simulink model "AOCS_m"  (R2023b)
settings: Solver=VariableStepAuto  StartTime=0.0  StopTime=100  MaxStep=0.01  RelTol=1e-4  AbsTol=1e-5
libraries: autolibbldc x3
settings Model: SimulationMode=accelerator  Creator=tiwan  LastModifiedBy=tiwan
settings SolverCC: AutoScaleAbsTol=off  InitialStep=0.01  ZeroCrossControl=EnableAll

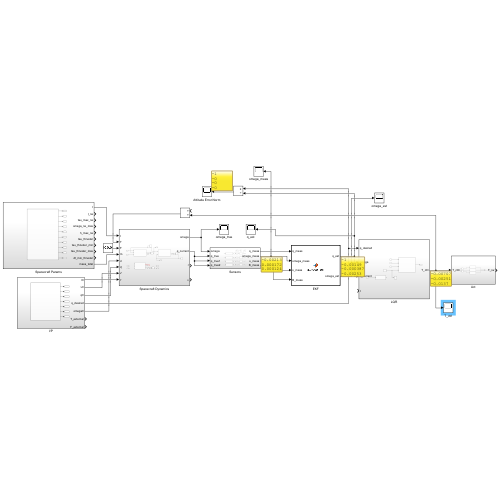
[thumbnail: Simulink's stored preview of the top-level diagram]
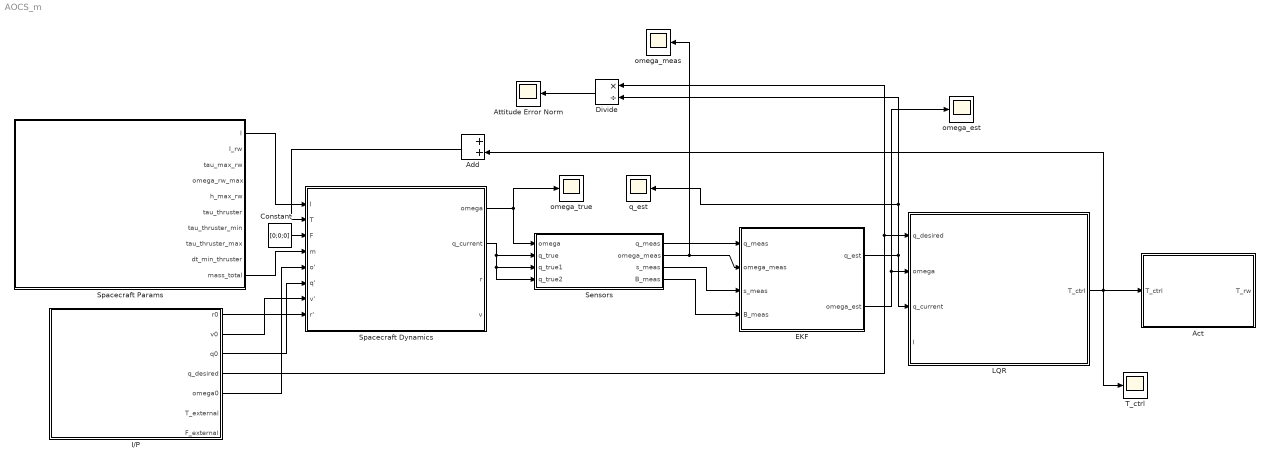
== system AOCS_m ==
  Act : Subsystem
  Add : Sum
  Attitude Error Norm : Scope
  Constant : Constant  Value=[0;0;0]
  Divide : Product  Inputs=*/
  EKF : MATLAB Function  TreatAsAtomicUnit=on
  I/P : Subsystem
  LQR : Subsystem
  Sensors : Subsystem
  Spacecraft Dynamics : Subsystem
  Spacecraft Params : Subsystem
  T_ctrl : Scope
  omega_est : Scope
  omega_meas : Scope
  omega_true : Scope
  q_est : Scope
  wires:
  Spacecraft Params/1(I) -> Spacecraft Dynamics/1(I)
  I/P/1(r0) -> Spacecraft Dynamics/8(r')
  I/P/2(v0) -> Spacecraft Dynamics/7(v')
  I/P/3(q0) -> Spacecraft Dynamics/6(q')
  I/P/5(omega0) -> Spacecraft Dynamics/5(o')
  I/P/4(q_desired) -> LQR/1(q_desired), Divide/1
  Spacecraft Dynamics/1(omega) -> Sensors/1(omega), omega_true/1
  Spacecraft Dynamics/2(q_current) -> Sensors/4(q_true2), Sensors/3(q_true1), Sensors/2(q_true)
  LQR/1(T_ctrl) -> Add/2, T_ctrl/1, Act/1(T_ctrl)
  Sensors/2(omega_meas) -> EKF/2(omega_meas), omega_meas/1
  Sensors/1(q_meas) -> EKF/1(q_meas)
  Sensors/3(s_meas) -> EKF/3(s_meas)
  Sensors/4(B_meas) -> EKF/4(B_meas)
  EKF/1(q_est) -> Divide/2, q_est/1, LQR/3(q_current)
  EKF/2(omega_est) -> LQR/2(omega), omega_est/1
  Spacecraft Params/10(mass_total) -> Spacecraft Dynamics/4(m)
  Constant/1 -> Spacecraft Dynamics/3(F)
  Divide/1 -> Attitude Error Norm/1
  Add/1 -> Spacecraft Dynamics/2(T)

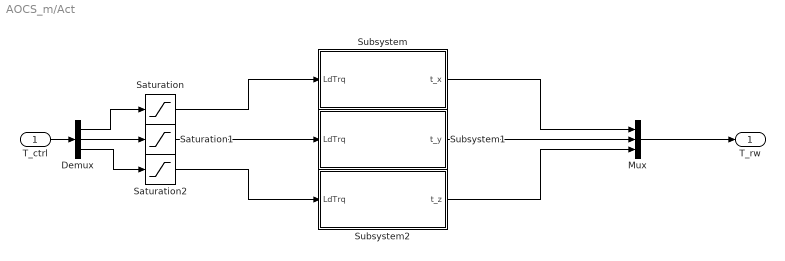
== system AOCS_m/Act ==
  T_ctrl : Inport
  Demux : Demux  Outputs=3
  Mux : Mux  Inputs=3
  Saturation : Saturate  UpperLimit=0.2  LowerLimit=-0.2
  Saturation1 : Saturate  UpperLimit=0.2  LowerLimit=-0.2
  Saturation2 : Saturate  UpperLimit=0.2  LowerLimit=-0.2
  Subsystem : Subsystem
  Subsystem1 : Subsystem
  Subsystem2 : Subsystem
  T_rw : Outport
  wires:
  T_ctrl/1 -> Demux/1
  Demux/1 -> Saturation/1
  Demux/2 -> Saturation1/1
  Demux/3 -> Saturation2/1
  Mux/1 -> T_rw/1
  Saturation/1 -> Subsystem/1(LdTrq)
  Saturation1/1 -> Subsystem1/1(LdTrq)
  Saturation2/1 -> Subsystem2/1(LdTrq)
  Subsystem1/1(t_y) -> Mux/2
  Subsystem/1(t_x) -> Mux/1
  Subsystem2/1(t_z) -> Mux/3

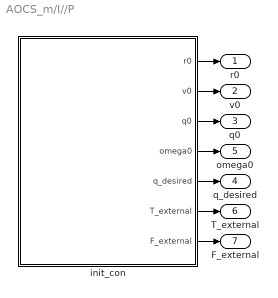
== system AOCS_m/I//P ==
  init_con : MATLAB Function  TreatAsAtomicUnit=on
  r0 : Outport
  v0 : Outport  Port=2
  q0 : Outport  Port=3
  q_desired : Outport  Port=4
  omega0 : Outport  Port=5
  T_external : Outport  Port=6
  F_external : Outport  Port=7
  wires:
  init_con/1(r0) -> r0/1
  init_con/7(F_external) -> F_external/1
  init_con/6(T_external) -> T_external/1
  init_con/5(q_desired) -> q_desired/1
  init_con/2(v0) -> v0/1
  init_con/3(q0) -> q0/1
  init_con/4(omega0) -> omega0/1

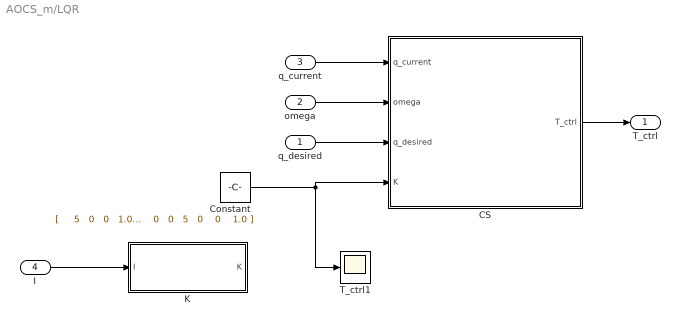
== system AOCS_m/LQR ==
  q_desired : Inport
  omega : Inport  Port=2
  q_current : Inport  Port=3
  I : Inport  Port=4
  CS : MATLAB Function  TreatAsAtomicUnit=on
  Constant : Constant  Value=|
      | [
      |     5   0   0   1.0  0    0;
      |     0   5   0   0    1.0  0;
      |     0   0   5   0    0    1.0
      | ]
  K : MATLAB Function  TreatAsAtomicUnit=on
  T_ctrl1 : Scope
  T_ctrl : Outport
  wires:
  q_desired/1 -> CS/3(q_desired)
  omega/1 -> CS/2(omega)
  q_current/1 -> CS/1(q_current)
  CS/1(T_ctrl) -> T_ctrl/1
  I/1 -> K/1(I)
  Constant/1 -> CS/4(K), T_ctrl1/1

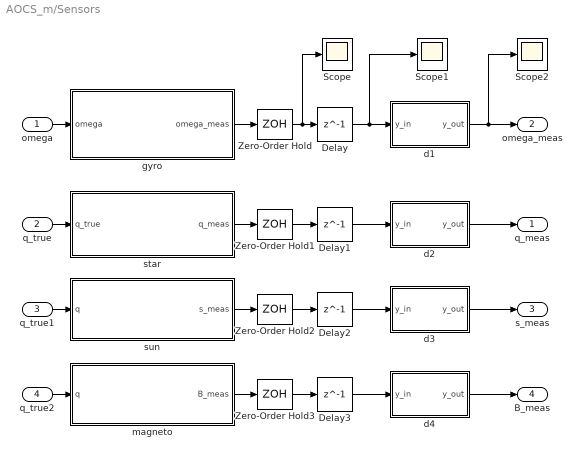
== system AOCS_m/Sensors ==
  omega : Inport
  q_true : Inport  Port=2
  q_true1 : Inport  Port=3
  q_true2 : Inport  Port=4
  Delay{,1..3} (4 alike) : Delay  DelayLength=1  InitialCondition=0  SampleTime=0.05
  Scope : Scope
  Scope1 : Scope
  Scope2 : Scope
  Zero-Order Hold : ZeroOrderHold  SampleTime=0.1
  Zero-Order Hold1 : ZeroOrderHold  SampleTime=-1
  Zero-Order Hold2 : ZeroOrderHold  SampleTime=-1
  Zero-Order Hold3 : ZeroOrderHold  SampleTime=-1
  d1 : MATLAB Function  TreatAsAtomicUnit=on
  d2 : MATLAB Function  TreatAsAtomicUnit=on
  d3 : MATLAB Function  TreatAsAtomicUnit=on
  d4 : MATLAB Function  TreatAsAtomicUnit=on
  gyro : MATLAB Function  TreatAsAtomicUnit=on
  magneto : MATLAB Function  TreatAsAtomicUnit=on
  star : MATLAB Function  TreatAsAtomicUnit=on
  sun : MATLAB Function  TreatAsAtomicUnit=on
  q_meas : Outport
  omega_meas : Outport  Port=2
  s_meas : Outport  Port=3
  B_meas : Outport  Port=4
  wires:
  omega/1 -> gyro/1(omega)
  q_true/1 -> star/1(q_true)
  star/1(q_meas) -> Zero-Order Hold1/1
  gyro/1(omega_meas) -> Zero-Order Hold/1
  Zero-Order Hold/1 -> Scope/1, Delay/1
  Zero-Order Hold1/1 -> Delay1/1
  Delay/1 -> Scope1/1, d1/1(y_in)
  Delay1/1 -> d2/1(y_in)
  d2/1(y_out) -> q_meas/1
  q_true1/1 -> sun/1(q)
  q_true2/1 -> magneto/1(q)
  magneto/1(B_meas) -> Zero-Order Hold3/1
  sun/1(s_meas) -> Zero-Order Hold2/1
  Zero-Order Hold2/1 -> Delay2/1
  Zero-Order Hold3/1 -> Delay3/1
  Delay2/1 -> d3/1(y_in)
  Delay3/1 -> d4/1(y_in)
  d3/1(y_out) -> s_meas/1
  d4/1(y_out) -> B_meas/1
  d1/1(y_out) -> Scope2/1, omega_meas/1

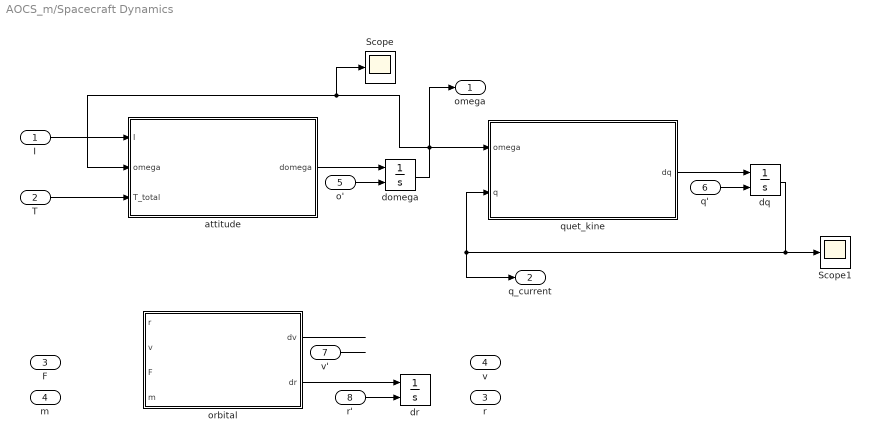
== system AOCS_m/Spacecraft Dynamics ==
  I : Inport
  T : Inport  Port=2
  F : Inport  Port=3
  m : Inport  Port=4
  o' : Inport  Port=5
  q' : Inport  Port=6
  v' : Inport  Port=7
  r' : Inport  Port=8
  Scope : Scope
  Scope1 : Scope
  attitude : MATLAB Function  TreatAsAtomicUnit=on
  domega : Integrator  InitialConditionSource=external
  dq : Integrator  InitialConditionSource=external
  dr : Integrator  InitialConditionSource=external
  orbital : MATLAB Function  TreatAsAtomicUnit=on
  quet_kine : MATLAB Function  TreatAsAtomicUnit=on
  omega : Outport
  q_current : Outport  Port=2
  r : Outport  Port=3
  v : Outport  Port=4
  wires:
  attitude/1(domega) -> domega/1
  domega/1 -> omega/1, Scope/1, attitude/2(omega), quet_kine/1(omega)
  quet_kine/1(dq) -> dq/1
  dq/1 -> Scope1/1, quet_kine/2(q), q_current/1
  orbital/1(dv) -> ?
  orbital/2(dr) -> dr/1
  I/1 -> attitude/1(I)
  T/1 -> attitude/3(T_total)
  o'/1 -> domega/2
  q'/1 -> dq/2
  v'/1 -> ?
  r'/1 -> dr/2

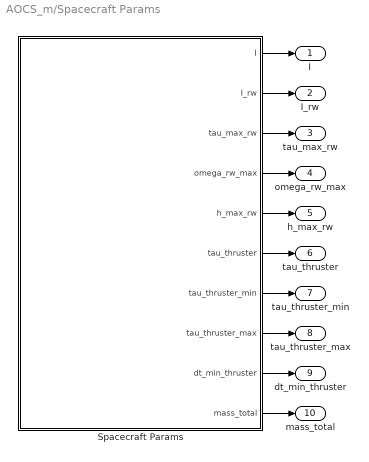
== system AOCS_m/Spacecraft Params ==
  Spacecraft Params : MATLAB Function  TreatAsAtomicUnit=on
  I : Outport
  I_rw : Outport  Port=2
  tau_max_rw : Outport  Port=3
  omega_rw_max : Outport  Port=4
  h_max_rw : Outport  Port=5
  tau_thruster : Outport  Port=6
  tau_thruster_min : Outport  Port=7
  tau_thruster_max : Outport  Port=8
  dt_min_thruster : Outport  Port=9
  mass_total : Outport  Port=10
  wires:
  Spacecraft Params/1(I) -> I/1
  Spacecraft Params/2(I_rw) -> I_rw/1
  Spacecraft Params/3(tau_max_rw) -> tau_max_rw/1
  Spacecraft Params/4(omega_rw_max) -> omega_rw_max/1
  Spacecraft Params/5(h_max_rw) -> h_max_rw/1
  Spacecraft Params/6(tau_thruster) -> tau_thruster/1
  Spacecraft Params/7(tau_thruster_min) -> tau_thruster_min/1
  Spacecraft Params/8(tau_thruster_max) -> tau_thruster_max/1
  Spacecraft Params/9(dt_min_thruster) -> dt_min_thruster/1
  Spacecraft Params/10(mass_total) -> mass_total/1

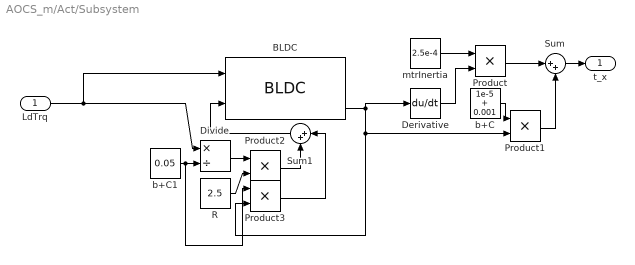
== system AOCS_m/Act/Subsystem ==
  LdTrq : Inport
  BLDC : autolibbldc/BLDC  VariantControl=pmsmVariant==pmsmEnum.TorqueInput  MechInput=Torque  SimType=Continuous  BlockSampleTime=25e-6  p=1  Rs=2.5  Ld=0.005  Lq=0.005  Lambda=0.0064  J=2.5e-4  B=2.6369e-06  F=0  Id_init=0  Iq_init=0  Th_init=0  Omega_init=0  RefBlkName='autolibbldc/BLDC'  aMode=5
      settings: LibrarySourceBlock=mcblib/Electrical Systems/Motors/BLDC
  Derivative : Derivative
  Divide : Product  Inputs=*/
  Product{,1..3} (4 alike) : Product
  R : Constant  Value=2.5
  Sum : Sum  Inputs=|++
  Sum1 : Sum  Inputs=|++
  b+C : Constant  Value=1e-5 + 0.001
  b+C1 : Constant  Value=0.05
  mtrInertia : Constant  Value=2.5e-4
  t_x : Outport
  wires:
  Product3/1 -> Sum1/1
  b+C1/1 -> Product3/1, Divide/2
  BLDC/3 -> Product3/2, Product1/2, Derivative/1
  LdTrq/1 -> Divide/1, BLDC/1
  R/1 -> Product2/2
  b+C/1 -> Product1/1
  Derivative/1 -> Product/2
  Sum1/1 -> BLDC/2
  mtrInertia/1 -> Product/1
  Product/1 -> Sum/1
  Divide/1 -> Product2/1
  Product1/1 -> Sum/2
  Product2/1 -> Sum1/2
  Sum/1 -> t_x/1

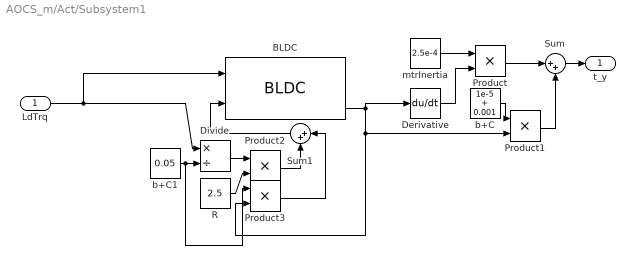
== system AOCS_m/Act/Subsystem1 ==
  LdTrq : Inport
  BLDC : autolibbldc/BLDC  VariantControl=pmsmVariant==pmsmEnum.TorqueInput  MechInput=Torque  SimType=Continuous  BlockSampleTime=25e-6  p=1  Rs=2.5  Ld=0.005  Lq=0.005  Lambda=0.0064  J=2.5e-4  B=2.6369e-06  F=0  Id_init=0  Iq_init=0  Th_init=0  Omega_init=0  RefBlkName='autolibbldc/BLDC'  aMode=5
      settings: LibrarySourceBlock=mcblib/Electrical Systems/Motors/BLDC
  Derivative : Derivative
  Divide : Product  Inputs=*/
  Product{,1..3} (4 alike) : Product
  R : Constant  Value=2.5
  Sum : Sum  Inputs=|++
  Sum1 : Sum  Inputs=|++
  b+C : Constant  Value=1e-5 + 0.001
  b+C1 : Constant  Value=0.05
  mtrInertia : Constant  Value=2.5e-4
  t_y : Outport
  wires:
  Product3/1 -> Sum1/1
  b+C1/1 -> Product3/1, Divide/2
  BLDC/3 -> Product3/2, Product1/2, Derivative/1
  LdTrq/1 -> Divide/1, BLDC/1
  R/1 -> Product2/2
  b+C/1 -> Product1/1
  Derivative/1 -> Product/2
  Sum1/1 -> BLDC/2
  mtrInertia/1 -> Product/1
  Product/1 -> Sum/1
  Divide/1 -> Product2/1
  Product1/1 -> Sum/2
  Product2/1 -> Sum1/2
  Sum/1 -> t_y/1

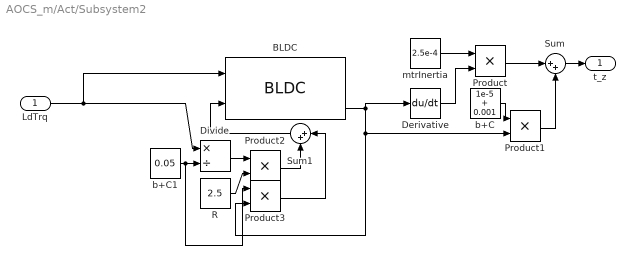
== system AOCS_m/Act/Subsystem2 ==
  LdTrq : Inport
  BLDC : autolibbldc/BLDC  VariantControl=pmsmVariant==pmsmEnum.TorqueInput  MechInput=Torque  SimType=Continuous  BlockSampleTime=25e-6  p=1  Rs=2.5  Ld=0.005  Lq=0.005  Lambda=0.0064  J=2.5e-4  B=2.6369e-06  F=0  Id_init=0  Iq_init=0  Th_init=0  Omega_init=0  RefBlkName='autolibbldc/BLDC'  aMode=5
      settings: LibrarySourceBlock=mcblib/Electrical Systems/Motors/BLDC
  Derivative : Derivative
  Divide : Product  Inputs=*/
  Product{,1..3} (4 alike) : Product
  R : Constant  Value=2.5
  Sum : Sum  Inputs=|++
  Sum1 : Sum  Inputs=|++
  b+C : Constant  Value=1e-5 + 0.001
  b+C1 : Constant  Value=0.05
  mtrInertia : Constant  Value=2.5e-4
  t_z : Outport
  wires:
  Product3/1 -> Sum1/1
  b+C1/1 -> Product3/1, Divide/2
  BLDC/3 -> Product3/2, Product1/2, Derivative/1
  LdTrq/1 -> Divide/1, BLDC/1
  R/1 -> Product2/2
  b+C/1 -> Product1/1
  Derivative/1 -> Product/2
  Sum1/1 -> BLDC/2
  mtrInertia/1 -> Product/1
  Product/1 -> Sum/1
  Divide/1 -> Product2/1
  Product1/1 -> Sum/2
  Product2/1 -> Sum1/2
  Sum/1 -> t_z/1

== matlab function AOCS_m/Sensors/d2 ==
  data: y_in input; y_out output
function y_out = dropout(y_in)
% Simulate dropout with 2% chance
if rand < 0.02
    y_out = zeros(size(y_in));  % Lost reading
else
    y_out = y_in;
end
end

== matlab function AOCS_m/Sensors/sun ==
  settings: updateMethod=DISCRETE
  data: q input; s_meas output
function s_meas = sun_sensor(q)
% Constants
s_inertial = [-1; 0; 0];           % Sun vector in inertial frame (unit vector)
noise_std = 0.01;                  % Sun sensor noise

% Convert quaternion to rotation matrix
q0 = q(1); qv = q(2:4);
q_cross = [    0   -qv(3)  qv(2);
            qv(3)     0   -qv(1);
           -qv(2)  qv(1)     0 ];
R = (q0^2 - qv' * qv) * eye(3) + 2 * (qv * qv') - 2 * q0 * q_cross;

% Transform Sun vector to body frame
s_body = R * s_inertial;

% Add noise
s_meas = s_body + noise_std * randn(3,1);
end

== matlab function AOCS_m/Sensors/magneto ==
  settings: updateMethod=DISCRETE
  data: q input; B_meas output
function B_meas = magnetometer(q)
% Constants
B_inertial = [0.2; -0.3; 0.4];     % Earth's magnetic field in inertial frame (μT)
noise_std = 0.01;                  % Magnetometer noise

% Convert quaternion to rotation matrix
q0 = q(1); qv = q(2:4);
q_cross = [    0   -qv(3)  qv(2);
            qv(3)     0   -qv(1);
           -qv(2)  qv(1)     0 ];
R = (q0^2 - qv' * qv) * eye(3) + 2 * (qv * qv') - 2 * q0 * q_cross;

% Transform magnetic field vector to body frame
B_body = R * B_inertial;

% Add noise
B_meas = B_body + noise_std * randn(3,1);
end

== matlab function AOCS_m/EKF ==
  data: q_meas input; q_est output; omega_meas input; s_meas input; B_meas input; omega_est output
function [q_est, omega_est] = attitude_ekf(q_meas, omega_meas, s_meas, B_meas)

% ======= Input Guards =======
if isempty(q_meas) || norm(q_meas) == 0 || any(isnan(q_meas))
    q_meas = [1; 0; 0; 0];  % fallback to identity quaternion
end

if isempty(omega_meas) || any(isnan(omega_meas))
    omega_meas = [0; 0; 0];
end

% ======= Persistent Variables =======
persistent x P
dt = 0.01;

if isempty(x)
    x = [q_meas; omega_meas];     % Initial state
    P = 1e-2 * eye(7);             % Initial covariance
end

% ======= Prediction Step =======
q = x(1:4);
omega = x(5:7);

% Quaternion derivative using Omega matrix
Omega = [0, -omega';
         omega, -skew(omega)];

q_dot = 0.5 * Omega * q;
q_pred = q + dt * q_dot;

% Normalize prediction
if norm(q_pred) == 0 || any(isnan(q_pred))
    q_pred = [1; 0; 0; 0];
else
    q_pred = q_pred / norm(q_pred);
end

omega_pred = omega;

% Jacobians (simplified)
F = eye(7);
Q = 1e-4 * eye(7);

x_pred = [q_pred; omega_pred];
P = F * P * F' + Q;

% ======= Measurement Update =======
H = eye(7);                 % Direct observation
R = 1e-3 * eye(7);           % Measurement noise

z = [q_meas; omega_meas];  % Measurement vector
z_pred = x_pred;           % Predicted measurement

% Kalman Gain
K = P * H' / (H * P * H' + R);

% EKF Update
x = x_pred + K * (z - z_pred);

% Normalize quaternion again
if norm(x(1:4)) == 0 || any(isnan(x(1:4)))
    x(1:4) = [1; 0; 0; 0];
else
    x(1:4) = x(1:4) / norm(x(1:4));
end

P = (eye(7) - K * H) * P;

% ======= Outputs =======
q_est = x(1:4);
omega_est = x(5:7);

end

% ======= Helper Function =======
function S = skew(w)
S = [ 0    -w(3)  w(2);
      w(3)  0    -w(1);
     -w(2)  w(1)  0   ];
end

== matlab function AOCS_m/Sensors/d3 ==
  data: y_in input; y_out output
function y_out = dropout(y_in)
% Simulate dropout with 2% chance
if rand < 0.02
    y_out = zeros(size(y_in));  % Lost reading
else
    y_out = y_in;
end
end

== matlab function AOCS_m/Sensors/d4 ==
  data: y_in input; y_out output
function y_out = dropout(y_in)
% Simulate dropout with 2% chance
if rand < 0.02
    y_out = zeros(size(y_in));  % Lost reading
else
    y_out = y_in;
end
end

== matlab function AOCS_m/LQR/K ==
  data: K output; I input
function K = computeK_manual(I)
% Fully Simulink-compatible LQR gain using Riccati iteration, no inv()

% Output definition
K = zeros(3,6);

% Validate input inertia
if any(size(I) ~= [3, 3])
    return;
end

% A, B matrices
A = [zeros(3), 0.5 * eye(3);
     zeros(3), zeros(3)];
B = [zeros(3);
     I \ eye(3)];  % Same as inv(I) * I_identity

% LQR weights
Q = diag([100, 100, 100, 5, 5, 5]);
R = 0.1 * eye(3);

% Riccati gradient descent
S = Q;
alpha = 1e-3;
max_iter = 500;
tol = 1e-4;

for i = 1:max_iter
    BT_S = B' * S;
    E = A' * S + S * A - S * B * (R \ BT_S) + Q;
    
    if norm(E, 'fro') < tol
        break;
    end
    
    S = S - alpha * E;
end

% Final LQR gain
K = R \ (B' * S);
end

== matlab function AOCS_m/Spacecraft Dynamics/attitude ==
  data: I input; domega output; omega input; T_total input
function domega = angular_dynamics(I, omega, T_total)
% Safety checks
if any(isnan(omega)) || any(isinf(omega))
    omega = [0;0;0];
end
if any(isnan(T_total)) || any(isinf(T_total))
    T_total = [0;0;0];
end

omega_cross = [  0        -omega(3)  omega(2);
              omega(3)     0       -omega(1);
             -omega(2)  omega(1)     0    ];

% Prevent singular matrix issues
if det(I) < 1e-6
    I = I + 1e-3 * eye(3);  % Regularize inertia
end

domega = I \ (T_total - omega_cross * (I * omega));
end

== matlab function AOCS_m/Spacecraft Params/Spacecraft Params ==
  data: I output; I_rw output; tau_max_rw output; omega_rw_max output; h_max_rw output; tau_thruster output; tau_thruster_min output; tau_thruster_max output; dt_min_thruster output; mass_total output
function [I, I_rw, tau_max_rw, omega_rw_max, h_max_rw, ...
          tau_thruster, tau_thruster_min, tau_thruster_max, ...
          dt_min_thruster, mass_total] = spacecraft_parameters()

% Spacecraft Moment of Inertia (kg·m²)
I = diag([2.5, 2.0, 1.8]);  % Customize per spacecraft

% Reaction Wheel Parameters
I_rw = [0.02; 0.02; 0.02];                    % Reaction wheel inertias
tau_max_rw = [0.1; 0.1; 0.1];                 % Max torque per RW (Nm)
omega_rw_max = [6000; 6000; 6000] * 2*pi/60;                  % Max RW speed (rad/s)
h_max_rw = I_rw .* omega_rw_max;             % Max angular momentum storage

% Thruster Parameters
tau_thruster = [0; 0; 0.5];      % Constant torque or command placeholder
tau_thruster_min = 0.01;         % Minimum on-time torque (Nm)
tau_thruster_max = 1.0;          % Max safe torque (Nm)
dt_min_thruster = 0.1;           % Min pulse time (s)

% Spacecraft Total Mass
mass_total = 50;  % kg

end

== matlab function AOCS_m/Spacecraft Dynamics/quet_kine ==
  data: omega input; dq output; q input
function dq = quaternion_kinematics(omega, q)
% omega: angular velocity [3x1]
% q: current quaternion [4x1]

Omega = [0       -omega(1) -omega(2) -omega(3);
         omega(1)  0        omega(3) -omega(2);
         omega(2) -omega(3) 0         omega(1);
         omega(3) omega(2) -omega(1)  0];

dq = 0.5 * Omega * q;
end

== matlab function AOCS_m/Spacecraft Dynamics/orbital ==
  data: r input; dv output; v input; F input; m input; dr output
function [dv, dr] = orbital_dynamics(r, v, F, m)
% r: position vector [3x1]
% v: velocity vector [3x1]
% F: total force applied [3x1]
% m: spacecraft mass (scalar)

mu = 398600.4418;  % Earth's gravitational parameter, km^3/s^2

% Two-body gravity + applied force
r_norm = norm(r);
a_gravity = -mu * r / r_norm^3;
a_applied = F / m;

dv = a_gravity + a_applied;
dr = v;
end

== matlab function AOCS_m/I//P/init_con ==
  data: r0 output; v0 output; q0 output; omega0 output; q_desired output; T_external output; F_external output
function [r0, v0, q0, omega0, q_desired, T_external, F_external] = initial_conditions()

% Initial orbital position (e.g., 700 km circular orbit in ECI frame)
r0 = [7000; 0; 0];          % km
v0 = [0; 7.5; 0];           % km/s (rough circular speed)

% Initial attitude (slightly off identity quaternion)
q0 = [0.999; 0.01; 0.01; 0.01];  % Should be normalized

% Initial angular velocity (rad/s)
omega0 = [0.01; 0.005; -0.01];   % Small rotation rate

% Desired attitude
q_desired = [1; 0; 0; 0];  % No rotation (identity quaternion)

% External disturbance torque (Nm)
T_external = [0.0001; 0.0001; 0.0002];

% External force (e.g., drag, solar radiation pressure) (N)
F_external = [0; 0; 0];  % Start with 0, can be added later

end

== matlab function AOCS_m/LQR/CS ==
  data: q_current input; T_ctrl output; omega input; q_desired input; K input
function T_ctrl = lqr_attitude_control(q_current, omega,q_desired, K)
% Inputs:
%   q_current: [4x1] current quaternion
%   omega:     [3x1] angular velocity
%   q_desired: [4x1] desired quaternion
%   K:         [3x6] LQR gain matrix

% Normalize quaternions (important for numerical stability)
q_current = q_current / norm(q_current);
q_desired = q_desired / norm(q_desired);

% Quaternion error: q_err = q_desired ⊗ q_current⁻¹
q_conj = [q_current(1); -q_current(2:4)];
q_err = quatmultiply(q_desired', q_conj')';  % result is 4x1

% Use only vector part of q_err (proportional part)
delta_q = q_err(2:4);  % 3x1

% LQR control law
x = [delta_q; omega];    % 6x1
T_ctrl = -K * x;         % 3x1 torque output

end

== matlab function AOCS_m/Sensors/gyro ==
  settings: updateMethod=DISCRETE
  data: omega input; omega_meas output
function omega_meas = gyro_sensor(omega)
% Simple gyroscope with bias and Gaussian noise
bias = [0.0005; -0.0003; 0.0004];     % Constant bias (rad/s)
noise_std = 0.001;                    % Noise std dev (rad/s)

omega_meas = omega + bias + noise_std * randn(3,1);
end

== matlab function AOCS_m/Sensors/star ==
  settings: updateMethod=DISCRETE
  data: q_true input; q_meas output
function q_meas = star_tracker(q_true)
% Star tracker with small attitude noise
noise_std = 0.002;

q_meas = q_true + noise_std * randn(4,1);
q_meas = q_meas / norm(q_meas);  % Normalize to unit quaternion
end

== matlab function AOCS_m/Sensors/d1 ==
  data: y_in input; y_out output
function y_out = dropout(y_in)
% Simulate dropout with 2% chance
if rand < 0.02
    y_out = zeros(size(y_in));  % Lost reading
else
    y_out = y_in;
end
end
